simulink library "SimulationLibrary"  (R2016b)
settings: Solver=ode45  StartTime=0.0  StopTime=10.0  RelTol=1e-3  EnableMultiTasking=on
values from neighbouring files (symbols this model uses):
  cassieEtherCatData = cassieEtherCat.getStructure    [simulationInitFcn.m]
  pelvisPosition = [0; 0; 1.01]    [simulationInitFcn.m]
undefined symbols (not defined in the file or in its folder): CassieParameters, leftFootDrive, leftLegMedulla, pelvisMedulla, X, Y, Z
libraries: sm_lib x86, SimulationLibrary x30, nesl_utility x18, Contact_Forces_Lib x2
(part 1 of 3)
settings Model: Creator=Mikhail  LastModifiedBy=Mikhail
settings DataIOCC: LimitDataPoints=on
settings OptimizationCC: LifeSpan=inf
settings DebuggingCC: AllowSymbolicDim=off  SFUnexpectedBacktrackingDiag=warning  SFNoUnconditionalDefaultTransitionDiag=warning  SFExecutionAtInitializationDiag=none
settings GRTTargetCC: TargetLangStandard=C89/C90 (ANSI)  GeneratePreprocessorConditionals=Disable all
settings ConfigComp: CovMetricSettings=dw  CovHtmlReporting=on  CovSaveCumulativeToWorkspaceVar=on  CovSaveSingleToWorkspaceVar=on  CovExternalEMLEnable=off

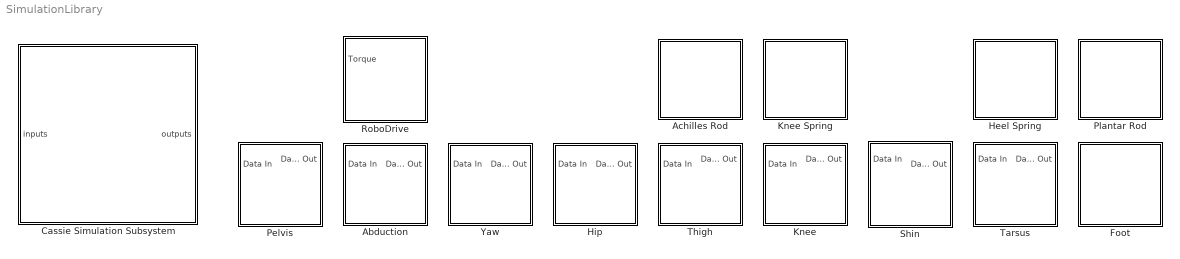
== system SimulationLibrary ==
  Abduction : Subsystem  mask{side=Left}
      mask init:
      | switch side
      |   case 1 % Left
      |     % Bus
      |     set_param([gcb, '/Bus Selector'], 'OutputSignals', 'leftAbductionDrive.outputs.torque');
      |     set_param([gcb, '/Bus Assignment'], 'AssignedSignals', 'leftAbductionDrive.inputs.position');
      |     
      |     % Solid
      |     set_param([gcb, '/Abduction'], 'ExtGeomFileName', 'left_abduction.stl');
      |     
      |     % Revolute Joint
      |     set_param([gcb, '/Revolute Joint'], 'PositionTargetValue', 'cassieEtherCatData.leftAbductionDrive.inputs.position');
      |     set_param([gcb, '/Revolute Joint'], 'DampingCoefficient', 'CassieParameters.motorViscousFrictionCoefficient(1)');
      |     
      |   case 2 % Right
      |     % Bus
      |     set_param([gcb, '/Bus Selector'], 'OutputSignals', 'rightAbductionDrive.outputs.torque');
      |     set_param([gcb, '/Bus Assignment'], 'AssignedSignals', 'rightAbductionDrive.inputs.position');
      |     
      |     % Solid
      |     set_param([gcb, '/Abduction'], 'ExtGeomFileName', 'right_abduction.stl');
      |     
      |     % Revolute Joint
      |     set_param([gcb, '/Revolute Joint'], 'PositionTargetValue', 'cassieEtherCatData.rightAbductionDrive.inputs.position');
      |     set_param([gcb, '/Revolute Joint'], 'DampingCoefficient', 'CassieParameters.motorViscousFrictionCoefficient(6)');
      | end % switch
      mask TypeOptions side: Left | Right
      mask Display: image('Cassie Abduction.png');
  Achilles Rod : Subsystem
      mask Display: image('Cassie Achilles Rod.png')
  Cassie Simulation Subsystem : Subsystem
      mask Display: image('Cassie.png');
  Foot : Subsystem  mask{side=Left}
      mask init:
      | switch side
      |   case 1 % Left
      |     % Solid
      |     set_param([gcb, '/Foot'], 'ExtGeomFileName', 'left_foot.stl');
      |     set_param([gcb, '/Foot'], 'CenterOfMass', '[4.74; 27.48; -0.14]/1000');
      |     set_param([gcb, '/Foot'], 'ProductsOfInertia', '[0.1716; -1.456; -98.63]/1000000');
      |     
      |     % Plantar
      |     set_param([gcb, '/Foot to Plantar Rod'], 'TranslationCartesianOffset', '[55; 0; 7.76]/1000');
      |     
      |     % Joint
      |     set_param([gcb, '/Revolute Joint'], 'PositionTargetValue', 'cassieEtherCatData.leftFootDrive.inputs.position');
      |     
      |   case 2 % Right
      |     % Solid
      |     set_param([gcb, '/Foot'], 'ExtGeomFileName', 'right_foot.stl');
      |     set_param([gcb, '/Foot'], 'CenterOfMass', '[4.74; 27.48; 0.14]/1000');
      |     set_param([gcb, '/Foot'], 'ProductsOfInertia', '[-0.1716; 1.456; -98.63]/1000000');
      |     
      |     % Plantar
      |     set_param([gcb, '/Foot to Plantar Rod'], 'TranslationCartesianOffset', '[55; 0; -7.76]/1000');
      |     
      |     % Joint
      |     set_param([gcb, '/Revolute Joint'], 'PositionTargetValue', 'cassieEtherCatData.rightFootDrive.inputs.position');
      | end % switch
      mask TypeOptions side: Left | Right
      mask Display: image('Cassie Foot.png');
  Heel Spring : Subsystem
  Hip : Subsystem  mask{side=Left}
      mask init:
      | switch side
      |   case 1 % Left
      |     % Bus
      |     set_param([gcb, '/Bus Selector'], 'OutputSignals', 'leftHipDrive.outputs.torque');
      |     set_param([gcb, '/Bus Assignment'], 'AssignedSignals', 'leftHipDrive.inputs.position');
      |     
      |     % Solid
      |     set_param([gcb, '/Hip'], 'ExtGeomFileName', 'left_hip.stl');
      |     set_param([gcb, '/Hip'], 'CenterOfMass', '[-55.72; 0; 0.01]/1000');
      |     set_param([gcb, '/Hip'], 'ProductsOfInertia', '[-0.04; -0.6251; 0.2462]/1000000');
      |     
      |     % Revolute Joint
      |     set_param([gcb, '/Revolute Joint'], 'PositionTargetValue', 'cassieEtherCatData.leftHipDrive.inputs.position');
      |     set_param([gcb, '/Revolute Joint'], 'DampingCoefficient', 'CassieParameters.motorViscousFrictionCoefficient(3)');
      |     
      |   case 2 % Right
      |     % Bus
      |     set_param([gcb, '/Bus Selector'], 'OutputSignals', 'rightHipDrive.outputs.torque');
      |     set_param([gcb, '/Bus Assignment'], 'AssignedSignals', 'rightHipDrive.inputs.position');
      |     
      |     % Solid
      |     set_param([gcb, '/Hip'], 'ExtGeomFileName', 'right_hip.stl');
      |     set_param([gcb, '/Hip'], 'CenterOfMass', '[-55.72; 0; -0.01]/1000');
      |     set_param([gcb, '/Hip'], 'ProductsOfInertia', '[0.04; 0.6251; 0.2462]/1000000');
      |     
      |     % Revolute Joint
      |     set_param([gcb, '/Revolute Joint'], 'PositionTargetValue', 'cassieEtherCatData.rightHipDrive.inputs.position');
      |     set_param([gcb, '/Revolute Joint'], 'DampingCoefficient', 'CassieParameters.motorViscousFrictionCoefficient(8)');
      | end % switch
      mask TypeOptions side: Left | Right
      mask Display: image('Cassie Hip.png');
  Knee : Subsystem  mask{side=Left}
      mask init:
      | switch side
      |   case 1 % Left
      |     % Bus
      |     set_param([gcb, '/Bus Selector'], 'OutputSignals', 'leftKneeDrive.outputs.torque');
      |     set_param([gcb, '/Bus Assignment'], 'AssignedSignals', 'leftKneeDrive.inputs.position');
      |     
      |     % Solid
      |     set_param([gcb, '/Knee'], 'ExtGeomFileName', 'left_knee.stl');
      |     set_param([gcb, '/Knee'], 'CenterOfMass', '[23.0; 32.07; -2.181]/1000');
      |     set_param([gcb, '/Knee'], 'ProductsOfInertia', '[0.739; 2.837; 956.4]/1000000');
      |     
      |     % Revolute Joint
      |     set_param([gcb, '/Revolute Joint'], 'PositionTargetValue', 'cassieEtherCatData.leftKneeDrive.inputs.position');
      |     set_param([gcb, '/Revolute Joint'], 'DampingCoefficient', 'CassieParameters.motorViscousFrictionCoefficient(4)');
      |     
      |   case 2 % Right
      |     % Bus
      |     set_param([gcb, '/Bus Selector'], 'OutputSignals', 'rightKneeDrive.outputs.torque');
      |     set_param([gcb, '/Bus Assignment'], 'AssignedSignals', 'rightKneeDrive.inputs.position');
      |     
      |     % Solid
      |     set_param([gcb, '/Knee'], 'ExtGeomFileName', 'right_knee.stl');
      |     set_param([gcb, '/Knee'], 'CenterOfMass', '[23.0; 32.07; 2.181]/1000');
      |     set_param([gcb, '/Knee'], 'ProductsOfInertia', '[-0.739; -2.837; 956.4]/1000000');
      |     
      |     % Revolute Joint
      |     set_param([gcb, '/Revolute Joint'], 'PositionTargetValue', 'cassieEtherCatData.rightKneeDrive.inputs.position');
      |     set_param([gcb, '/Revolute Joint'], 'DampingCoefficient', 'CassieParameters.motorViscousFrictionCoefficient(9)');
      | end % switch
      mask TypeOptions side: Left | Right
      mask Display: image('Cassie Knee.png');
  Knee Spring : Subsystem
  Pelvis : Subsystem
      mask Display: image('Cassie Pelvis.png');
  Plantar Rod : Subsystem
      mask Display: image('Cassie Plantar Rod.png')
  RoboDrive : Subsystem  mask{model=115x25}
      mask prompts: model "RoboDrive model:"
      mask init:
      | switch model
      |   case 1 % 115x25
      |     set_param([gcb '/Peak Torque'], 'Value', '12.2');
      |     set_param([gcb '/Peak Speed'], 'Value', '1300*2*pi/60');
      |     set_param([gcb '/Rotor'], 'MomentsOfInertia', '[0 0 365]/1000000');
      |   case 2 % 85x13
      |     set_param([gcb '/Peak Torque'], 'Value', '4.5');
      |     set_param([gcb '/Peak Speed'], 'Value', '2900*2*pi/60');
      |     set_param([gcb '/Rotor'], 'MomentsOfInertia', '[0 0 61]/1000000');
      |   case 3 % 50x8
      |     set_param([gcb '/Peak Torque'], 'Value', '0.9');
      |     set_param([gcb '/Peak Speed'], 'Value', '5500*2*pi/60');
      |     set_param([gcb '/Rotor'], 'MomentsOfInertia', '[0 0 4.9]/1000000');
      | end % switch
      mask TypeOptions model: 115x25 | 85x13 | 50x8
      mask Display: image('RoboDrive.png')
  Shin : Subsystem  mask{side=Left}
      mask init:
      | switch side
      |   case 1 % Left
      |     % Bus
      |     set_param([gcb, '/Bus Assignment'], 'AssignedSignals', 'leftLegMedulla.miscInputs.kneeSpringEncoder');
      |     
      |     % Solid
      |     set_param([gcb, '/Shin'], 'ExtGeomFileName', 'left_shin.stl');
      |     set_param([gcb, '/Shin'], 'CenterOfMass', '[183.38; 1.169; 0.2123]/1000');
      |     set_param([gcb, '/Shin'], 'ProductsOfInertia', '[0.2652; -0.1941; 333.5]/1000000');
      |     
      |   case 2 % Right
      |     % Bus
      |     set_param([gcb, '/Bus Assignment'], 'AssignedSignals', 'rightLegMedulla.miscInputs.kneeSpringEncoder');
      |     
      |     % Solid
      |     set_param([gcb, '/Shin'], 'ExtGeomFileName', 'right_shin.stl');
      |     set_param([gcb, '/Shin'], 'CenterOfMass', '[183.38; 1.169; -0.2123]/1000');
      |     set_param([gcb, '/Shin'], 'ProductsOfInertia', '[-0.2652; 0.1941; 333.5]/1000000');
      | end % switch
      mask TypeOptions side: Left | Right
      mask Display: image('Cassie Shin.png');
  Tarsus : Subsystem  mask{side=Left}
      mask init:
      | switch side
      |   case 1 % Left
      |     % Bus
      |     set_param([gcb, '/Bus Selector'], 'OutputSignals', 'leftFootDrive.outputs.torque');
      |     set_param([gcb, '/Bus Assignment'], 'AssignedSignals', 'leftFootDrive.inputs.position,leftLegMedulla.miscInputs.ankleJointEncoder');
      |     
      |     % Solid
      |     set_param([gcb, '/Tarsus'], 'ExtGeomFileName', 'left_tarsus.stl');
      |     set_param([gcb, '/Tarsus'], 'CenterOfMass', '[110.46; -30.58; -1.31]/1000');
      |     set_param([gcb, '/Tarsus'], 'ProductsOfInertia', '[36.15; -63.29; -2878]/1000000');
      |     
      |     % Transforms
      |     set_param([gcb, '/Tarsus to Foot Drive'], 'TranslationCartesianOffset', '[58 -34 22.75]/1000');
      |     set_param([gcb, '/Tarsus to Spring'], 'TranslationCartesianOffset', '[-12.69 -30.59 0.92]/1000');
      |     set_param([gcb, '/Tarsus to Spring'], 'RotationSequenceAngles', '[155.8, 0.315, 4.47]');
      |     set_param([gcb, '/Foot Crank to Plantar Rod'], 'TranslationCartesianOffset', '[55 0 -7.91]/1000');
      |     set_param([gcb, '/Foot Crank Transform'], 'RotationAngle', '0');
      |     
      |     % Revolute Joint
      |     set_param([gcb, '/Foot Crank Revolute Joint'], 'PositionTargetValue', 'cassieEtherCatData.leftFootDrive.inputs.position');
      |     set_param([gcb, '/Foot Crank Revolute Joint'], 'DampingCoefficient', 'CassieParameters.motorViscousFrictionCoefficient(5)');
      |     
      |   case 2 % Right
      |     % Bus
      |     set_param([gcb, '/Bus Selector'], 'OutputSignals', 'rightFootDrive.outputs.torque');
      |     set_param([gcb, '/Bus Assignment'], 'AssignedSignals', 'rightFootDrive.inputs.position,rightLegMedulla.miscInputs.ankleJointEncoder');
      |     
      |     % Solid
      |     set_param([gcb, '/Tarsus'], 'ExtGeomFileName', 'right_tarsus.stl');
      |     set_param([gcb, '/Tarsus'], 'CenterOfMass', '[110.46; -30.58; 1.31]/1000');
      |     set_param([gcb, '/Tarsus'], 'ProductsOfInertia', '[-36.15; 63.29; -2878]/1000000');
      |     
      |     % Transforms
      |     set_param([gcb, '/Tarsus to Foot Drive'], 'TranslationCartesianOffset', '[58 -34 -22.75]/1000');
      |     set_param([gcb, '/Tarsus to Spring'], 'TranslationCartesianOffset', '[-12.69 -30.59 -0.92]/1000');
      |     set_param([gcb, '/Tarsus to Spring'], 'RotationSequenceAngles', '[155.8, -0.315, -4.47]');
      |     set_param([gcb, '/Foot Crank to Plantar Rod'], 'TranslationCartesianOffset', '[55 0 7.91]/1000');
      |     set_param([gcb, '/Foot Crank Transform'], 'RotationAngle', 'pi');
      |     
      |     % Revolute Joint
      |     set_param([gcb, '/Foot Crank Revolute Joint'], 'PositionTargetValue', 'cassieEtherCatData.rightFootDrive.inputs.position');
      |     set_param([gcb, '/Foot Crank Revolute Joint'], 'DampingCoefficient', 'CassieParameters.motorViscousFrictionCoefficient(10)');
      | end % switch
      mask TypeOptions side: Left | Right
      mask Display: image('Cassie Tarsus.png');
  Thigh : Subsystem  mask{side=Left}
      mask init:
      | switch side
      |   case 1 % Left
      |     % Solid
      |     set_param([gcb, '/Thigh'], 'ExtGeomFileName', 'left_thigh.stl');
      |     set_param([gcb, '/Thigh'], 'CenterOfMass', '[59.46; 0.05; -35.81]/1000');
      |     set_param([gcb, '/Thigh'], 'ProductsOfInertia', '[-19.26; -11685; 283.6]/1000000');
      |     
      |     % Knee
      |     set_param([gcb, '/Thigh to Knee'], 'TranslationCartesianOffset', '[0.12, 0, 0.0045]');
      |     
      |     % Achilles
      |     set_param([gcb, '/Thigh to Achilles'], 'TranslationCartesianOffset', '[0, 0, 0.045]');
      |     
      |   case 2 % Right
      |     % Solid
      |     set_param([gcb, '/Thigh'], 'ExtGeomFileName', 'right_thigh.stl');
      |     set_param([gcb, '/Thigh'], 'CenterOfMass', '[59.46; 0.05; 35.81]/1000');
      |     set_param([gcb, '/Thigh'], 'ProductsOfInertia', '[19.26; 11685; 283.6]/1000000');
      |     
      |     % Knee
      |     set_param([gcb, '/Thigh to Knee'], 'TranslationCartesianOffset', '[0.12, 0, -0.0045]');
      |     
      |     % Achilles
      |     set_param([gcb, '/Thigh to Achilles'], 'TranslationCartesianOffset', '[0, 0, -0.045]');
      | end % switch
      mask TypeOptions side: Left | Right
      mask Display: image('Cassie Thigh.png');
  Yaw : Subsystem  mask{side=Left}
      mask init:
      | switch side
      |   case 1 % Left
      |     % Bus
      |     set_param([gcb, '/Bus Selector'], 'OutputSignals', 'leftYawDrive.outputs.torque');
      |     set_param([gcb, '/Bus Assignment'], 'AssignedSignals', 'leftYawDrive.inputs.position');
      |     
      |     % Solid
      |     set_param([gcb, '/Yaw'], 'ExtGeomFileName', 'left_yaw.stl');
      |     set_param([gcb, '/Yaw'], 'CenterOfMass', '[25.7; 0.1; 17.93]/1000');
      |     set_param([gcb, '/Yaw'], 'ProductsOfInertia', '[2.61; 1.53; 0.703]/1000000');
      |     
      |     % Revolute Joint
      |     set_param([gcb, '/Revolute Joint'], 'PositionTargetValue', 'cassieEtherCatData.leftYawDrive.inputs.position');
      |     set_param([gcb, '/Revolute Joint'], 'DampingCoefficient', 'CassieParameters.motorViscousFrictionCoefficient(2)');
      |     
      |   case 2 % Right
      |     % Bus
      |     set_param([gcb, '/Bus Selector'], 'OutputSignals', 'rightYawDrive.outputs.torque');
      |     set_param([gcb, '/Bus Assignment'], 'AssignedSignals', 'rightYawDrive.inputs.position');
      |     
      |     % Solid
      |     set_param([gcb, '/Yaw'], 'ExtGeomFileName', 'right_yaw.stl');
      |     set_param([gcb, '/Yaw'], 'CenterOfMass', '[25.7; -0.1; 17.93]/1000');
      |     set_param([gcb, '/Yaw'], 'ProductsOfInertia', '[-2.61; 1.53; -0.703]/1000000');
      |     
      |     % Revolute Joint
      |     set_param([gcb, '/Revolute Joint'], 'PositionTargetValue', 'cassieEtherCatData.rightYawDrive.inputs.position');
      |     set_param([gcb, '/Revolute Joint'], 'DampingCoefficient', 'CassieParameters.motorViscousFrictionCoefficient(7)');
      | end % switch
      mask TypeOptions side: Left | Right
      mask Display: image('Cassie Yaw.png');

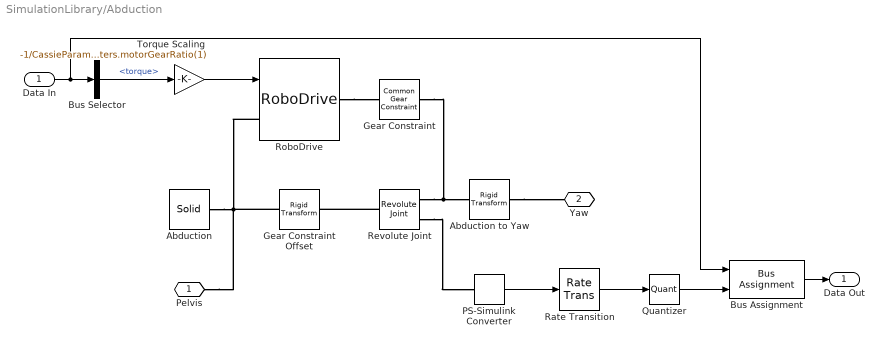
== system SimulationLibrary/Abduction ==
  Data In : Inport  OutDataTypeStr=Bus: cassieEtherCatBus
  Abduction : sm_lib/Body Elements/Solid  InertiaType=Custom  Mass=0  MassUnits=kg  CenterOfMass=[0; 0; 0]  CenterOfMassUnits=m  MomentsOfInertia=[0; 0; 0]  MomentsOfInertiaUnits=kg*m^2  ProductsOfInertia=[0; 0; 0]  ProductsOfInertiaUnits=kg*m^2  DensityBased=on  Density=1000  DensityUnits=kg/(m^3)  DoExposeReferenceFrame=on  SerializedFrames=<Frames/>  GraphicType=FromGeometry  MarkerShape=Sphere  MarkerSize=10  MarkerSizeUnits=m  GraphicVisPropType=AdvancedVisualProperties  GraphicDiffuseColor=simulationParameters.diffuseColor  GraphicSpecularColor=simulationParameters.specularColor  GraphicAmbientColor=simulationParameters.ambientColor  GraphicEmissiveColor=simulationParameters.emissiveColor  GraphicShininess=simulationParameters.shininess  GraphicOpacity=1  GeometryShape=FromFile  RectangleSize=[1 1]  RectangleSizeUnits=m  BrickDimensions=[0.15 0.15 0.2]  BrickDimensionUnits=m  CylinderRadius=0.05  CylinderRadiusUnits=m  CylinderLength=0.1  CylinderLengthUnits=m  SphereRadius=1  SphereRadiusUnits=m  EllipsoidRadii=[1 1 1]  EllipsoidRadiiUnits=m  ExtrusionCrossSection=[1 1; -1 1; -1 -1; 1 -1]  ExtrusionCrossSectionUnits=m  ExtrusionLength=1  ExtrusionLengthUnits=m  PolygonNumSides=3  PolygonOuterRadius=1  PolygonOuterRadiusUnits=m  ExtGeomFileType=STL  ExtGeomFileName=left_abduction.stl  ExtGeomFileUnits=m  RevolutionCrossSection=[1 1; 1 -1; 2 -1; 2 1]  RevolutionCrossSectionUnits=m  RevolutionExtent=Full  RevolutionAngle=180  RevolutionAngleUnits=deg
  Abduction to Yaw : sm_lib/Frames and Transforms/Rigid Transform  TranslationMethod=Cartesian  TranslationStandardOffset=0  TranslationLengthUnit=m  TranslationStandardAxis=+Z  TranslationCartesianOffset=[0, 0, -0.07]  TranslationROffset=0  TranslationROffsetUnits=m  TranslationZOffset=0  TranslationZOffsetUnits=m  TranslationThetaOffset=0  TranslationThetaOffsetUnits=deg  RotationMethod=RotationMatrix  RotationAngleUnits=deg  RotationStandardAxis=+Z  RotationAngle=0.0  RotationArbitraryAxis=[0 0 1]  FollAlignAxisA=+X  BaseAlignAxisA=+Y  FollAlignAxisB=+Y  BaseAlignAxisB=+Z  RotationSequenceAxes=FollowerAxes  RotationSequence=XYZ  RotationSequenceAngles=[90 0 0]  RotationSequenceAnglesUnits=deg  RotationMatrix=[0, 0, -1; 0, 1, 0; 1, 0, 0]
  Bus Assignment : BusAssignment  AssignedSignals=leftAbductionDrive.inputs.position
  Bus Selector : BusSelector  OutputSignals=leftAbductionDrive.outputs.torque
  Gear Constraint : sm_lib/Gears and Couplings/Gears/Common Gear Constraint  GearType=External  SpecificationType=CenterDistanceRatio  CenterDistance=1e-6  CenterDistanceUnits=m  GearRatio=CassieParameters.motorGearRatio(1)  BaseGearRadius=10.0  BaseGearRadiusUnits=cm  FollGearRadius=10.0  FollGearRadiusUnits=cm  AssemblyGearRotation=Free
  Gear Constraint Offset : sm_lib/Frames and Transforms/Rigid Transform  TranslationMethod=StandardAxis  TranslationStandardOffset=1e-6  TranslationLengthUnit=m  TranslationStandardAxis=+Y  TranslationCartesianOffset=[0 0 0]  TranslationROffset=0  TranslationROffsetUnits=m  TranslationZOffset=0  TranslationZOffsetUnits=m  TranslationThetaOffset=0  TranslationThetaOffsetUnits=deg  RotationMethod=None  RotationAngleUnits=deg  RotationStandardAxis=+Z  RotationAngle=0.0  RotationArbitraryAxis=[0 0 1]  FollAlignAxisA=+X  BaseAlignAxisA=+Y  FollAlignAxisB=+Y  BaseAlignAxisB=+Z  RotationSequenceAxes=FollowerAxes  RotationSequence=XYX  RotationSequenceAngles=[0 0 0]  RotationSequenceAnglesUnits=deg  RotationMatrix=[1 0 0; 0 1 0; 0 0 1]
  PS-Simulink Converter : nesl_utility/PS-Simulink Converter  PhysicalDomain=network_engine_domain  SubClassName=ps_output  LeftPortType=input  RightPortType=output  PseudoPeriodic=off  Frequencies=[]  Unit=rad  AffineConversion=off
  Quantizer : Quantizer  QuantizationInterval=(2*pi)/(CassieParameters.motorEncoderTicks(1)*CassieParameters.motorGearRatio(1))
  Rate Transition : RateTransition  Deterministic=off  OutPortSampleTime=CassieParameters.etherCatSampleTime
  Revolute Joint : sm_lib/Joints/Revolute Joint  SenseConstraintForce=off  SenseConstraintForceX=off  SenseConstraintForceY=off  SenseConstraintForceZ=off  SenseConstraintTorque=off  SenseConstraintTorqueX=off  SenseConstraintTorqueY=off  SenseConstraintTorqueZ=off  SenseTotalForce=off  SenseTotalForceX=off  SenseTotalForceY=off  SenseTotalForceZ=off  SenseTotalTorque=off  SenseTotalTorqueX=off  SenseTotalTorqueY=off  SenseTotalTorqueZ=off  CompositeWrenchDir=FollowerOnBase  CompositeWrenchFrame=BaseFrame  EquilibriumPosition=0  EquilibriumPositionUnits=rad  SpringStiffness=0  SpringStiffnessUnits=N*m/rad  DampingCoefficient=CassieParameters.motorViscousFrictionCoefficient(1)  DampingCoefficientUnits=N*m/(rad/s)  TorqueActuationMode=NoTorque  MotionActuationMode=ComputedMotion  SensePosition=on  SenseVelocity=off  SenseAcceleration=off  SenseTorqueForce=off  PositionTargetSpecify=on  PositionTargetPriority=High  PositionTargetValue=cassieEtherCatData.leftAbductionDrive.inputs.position  PositionTargetValueUnits=rad  VelocityTargetSpecify=on  VelocityTargetPriority=High  VelocityTargetValue=0  VelocityTargetValueUnits=rad/s
  RoboDrive : SimulationLibrary/RoboDrive  model=85x13
  Torque Scaling : Gain  Gain=-1/CassieParameters.motorGearRatio(1)
  Pelvis : PMIOPort  Port=1  Side=Left
  Yaw : PMIOPort  Port=2  Side=Right
  Data Out : Outport
  wires:
  Torque Scaling/1 -> RoboDrive/1
  Data In/1 -> Bus Selector/1, Bus Assignment/1
  Bus Assignment/1 -> Data Out/1
  Rate Transition/1 -> Quantizer/1
  Bus Selector/1 -> Torque Scaling/1  "<torque>"
  PS-Simulink Converter/1 -> Rate Transition/1
  Quantizer/1 -> Bus Assignment/2
  connections:
  Pelvis/RConn1 -- RoboDrive/LConn1 -- Abduction/RConn1 -- Gear Constraint Offset/LConn1
  Revolute Joint/LConn1 -- Gear Constraint Offset/RConn1
  RoboDrive/RConn1 -- Gear Constraint/LConn1
  Revolute Joint/RConn1 -- Abduction to Yaw/LConn1 -- Gear Constraint/RConn1
  Revolute Joint/RConn2 -- PS-Simulink Converter/LConn1
  Abduction to Yaw/RConn1 -- Yaw/RConn1

== system SimulationLibrary/Achilles Rod ==
  Achilles Rod : sm_lib/Body Elements/Solid  Commented=on  InertiaType=Custom  Mass=0.1567  MassUnits=kg  CenterOfMass=[247.19; 0; 0]/1000  CenterOfMassUnits=m  MomentsOfInertia=[3.7538; 14061; 14061]/1000000  MomentsOfInertiaUnits=kg*m^2  ProductsOfInertia=[0; 0.0082; 0.0068]/1000000  ProductsOfInertiaUnits=kg*m^2  DensityBased=on  Density=1000  DensityUnits=kg/(m^3)  DoExposeReferenceFrame=on  SerializedFrames=<Frames/>  GraphicType=FromGeometry  MarkerShape=Sphere  MarkerSize=10  GraphicVisPropType=AdvancedVisualProperties  GraphicDiffuseColor=simulationParameters.diffuseColor  GraphicSpecularColor=simulationParameters.specularColor  GraphicAmbientColor=simulationParameters.ambientColor  GraphicEmissiveColor=simulationParameters.emissiveColor  GraphicShininess=simulationParameters.shininess  GraphicOpacity=1.0  GeometryShape=FromFile  RectangleSize=[1 1]  RectangleSizeUnits=m  BrickDimensions=[1 1 1]  BrickDimensionUnits=m  CylinderRadius=1  CylinderRadiusUnits=m  CylinderLength=1  CylinderLengthUnits=m  SphereRadius=1  SphereRadiusUnits=m  EllipsoidRadii=[1 1 1]  EllipsoidRadiiUnits=m  ExtrusionCrossSection=[1 1; -1 1; -1 -1; 1 -1]  ExtrusionCrossSectionUnits=m  ExtrusionLength=1  ExtrusionLengthUnits=m  PolygonNumSides=3  PolygonOuterRadius=1  PolygonOuterRadiusUnits=m  ExtGeomFileType=STL  ExtGeomFileName=achilles_rod.stl  ExtGeomFileUnits=m  RevolutionCrossSection=[1 1; 1 -1; 2 -1; 2 1]  RevolutionCrossSectionUnits=m  RevolutionExtent=Full  RevolutionAngle=180  RevolutionAngleUnits=deg
  Distance Constraint : sm_lib/Constraints/Distance Constraint  Distance=0.5012  DistanceUnits=m  SenseSignedForceMagnitude=off  SenseTorque=off  SenseForce=off  WrenchDir=FollowerOnBase  WrenchFrame=BaseFrame
  Rigid Transform : sm_lib/Frames and Transforms/Rigid Transform  Commented=on  TranslationMethod=Cartesian  TranslationStandardOffset=50.14  TranslationLengthUnit=m  TranslationStandardAxis=+Z  TranslationCartesianOffset=[0.5012 0 0]  TranslationROffset=0  TranslationROffsetUnits=m  TranslationZOffset=0  TranslationZOffsetUnits=m  TranslationThetaOffset=0  TranslationThetaOffsetUnits=deg  RotationMethod=None  RotationAngleUnits=deg  RotationStandardAxis=+Z  RotationAngle=0.0  RotationArbitraryAxis=[0 0 1]  FollAlignAxisA=+X  BaseAlignAxisA=+Y  FollAlignAxisB=+Y  BaseAlignAxisB=+Z  RotationSequenceAxes=FollowerAxes  RotationSequence=XYX  RotationSequenceAngles=[0 0 0]  RotationSequenceAnglesUnits=deg  RotationMatrix=[1 0 0; 0 1 0; 0 0 1]
  Spring Spherical Joint : sm_lib/Joints/Spherical Joint  Commented=on  SenseConstraintForce=off  SenseConstraintForceX=off  SenseConstraintForceY=off  SenseConstraintForceZ=off  SenseConstraintTorque=off  SenseConstraintTorqueX=off  SenseConstraintTorqueY=off  SenseConstraintTorqueZ=off  SenseTotalForce=off  SenseTotalForceX=off  SenseTotalForceY=off  SenseTotalForceZ=off  SenseTotalTorque=off  SenseTotalTorqueX=off  SenseTotalTorqueY=off  SenseTotalTorqueZ=off  CompositeWrenchDir=FollowerOnBase  CompositeWrenchFrame=BaseFrame  DefPosRotationMethod=None  DefPosRotationAngleUnits=deg  DefPosRotationStandardAxis=+Z  DefPosRotationAngle=0.0  DefPosRotationArbitraryAxis=[0 0 1]  DefPosFollAlignAxisA=+X  DefPosBaseAlignAxisA=+Y  DefPosFollAlignAxisB=+Y  DefPosBaseAlignAxisB=+Z  DefPosRotationSequenceAxes=FollowerAxes  DefPosRotationSequence=XYX  DefPosRotationSequenceAngles=[0 0 0]  DefPosRotationSequenceAnglesUnits=deg  DefPosRotationMatrix=[1 0 0; 0 1 0; 0 0 1]  EqPosRotationMethod=None  EqPosRotationAngleUnits=deg  EqPosRotationStandardAxis=+Z  EqPosRotationAngle=0.0  EqPosRotationArbitraryAxis=[0 0 1]  EqPosFollAlignAxisA=+X  EqPosBaseAlignAxisA=+Y  EqPosFollAlignAxisB=+Y  EqPosBaseAlignAxisB=+Z  EqPosRotationSequenceAxes=FollowerAxes  EqPosRotationSequence=XYX  EqPosRotationSequenceAngles=[0 0 0]  EqPosRotationSequenceAnglesUnits=deg  EqPosRotationMatrix=[1 0 0; 0 1 0; 0 0 1]  SpringStiffness=0  SpringStiffnessUnits=N*m/deg  DampingCoefficient=0  DampingCoefficientUnits=N*m/(deg/s)  ActuateTorqueX=off  ActuateTorqueY=off  ActuateTorqueZ=off  ActuateTorque=off  TorqueActuationMode=NoTorque  MotionActuationMode=ComputedMotion  ActuationFrame=BaseFrame  SensePosition=off  SenseVelocityX=off  SenseVelocityY=off  SenseVelocityZ=off  SenseVelocity=off  SenseAccelerationX=off  SenseAccelerationY=off  SenseAccelerationZ=off  SenseAcceleration=off  SenseTorqueX=off  SenseTorqueY=off  SenseTorqueZ=off  SenseTorqueForce=off  SensingFrame=BaseFrame  PositionTargetRotationMethod=None  PositionTargetRotationAngleUnits=deg  PositionTargetRotationStandardAxis=+Z  PositionTargetRotationAngle=0.0  PositionTargetRotationArbitraryAxis=[0 0 1]  PositionTargetFollAlignAxisA=+X  PositionTargetBaseAlignAxisA=+Y  PositionTargetFollAlignAxisB=+Y  PositionTargetBaseAlignAxisB=+Z  PositionTargetRotationSequenceAxes=FollowerAxes  PositionTargetRotationSequence=XYX  PositionTargetRotationSequenceAngles=[0 0 0]  PositionTargetRotationSequenceAnglesUnits=deg  PositionTargetRotationMatrix=[1 0 0; 0 1 0; 0 0 1]  PositionTargetSpecify=off  PositionTargetPriority=High  VelocityTargetValue=[0 0 0]  VelocityTargetValueUnits=deg/s  VelocityTargetSpecify=off  VelocityTargetPriority=High  VelocityTargetInFollowerFrame=on
  Thigh Spherical Joint : sm_lib/Joints/Spherical Joint  Commented=on  SenseConstraintForce=off  SenseConstraintForceX=off  SenseConstraintForceY=off  SenseConstraintForceZ=off  SenseConstraintTorque=off  SenseConstraintTorqueX=off  SenseConstraintTorqueY=off  SenseConstraintTorqueZ=off  SenseTotalForce=off  SenseTotalForceX=off  SenseTotalForceY=off  SenseTotalForceZ=off  SenseTotalTorque=off  SenseTotalTorqueX=off  SenseTotalTorqueY=off  SenseTotalTorqueZ=off  CompositeWrenchDir=FollowerOnBase  CompositeWrenchFrame=BaseFrame  DefPosRotationMethod=None  DefPosRotationAngleUnits=deg  DefPosRotationStandardAxis=+Z  DefPosRotationAngle=0.0  DefPosRotationArbitraryAxis=[0 0 1]  DefPosFollAlignAxisA=+X  DefPosBaseAlignAxisA=+Y  DefPosFollAlignAxisB=+Y  DefPosBaseAlignAxisB=+Z  DefPosRotationSequenceAxes=FollowerAxes  DefPosRotationSequence=XYX  DefPosRotationSequenceAngles=[0 0 0]  DefPosRotationSequenceAnglesUnits=deg  DefPosRotationMatrix=[1 0 0; 0 1 0; 0 0 1]  EqPosRotationMethod=None  EqPosRotationAngleUnits=deg  EqPosRotationStandardAxis=+Z  EqPosRotationAngle=0.0  EqPosRotationArbitraryAxis=[0 0 1]  EqPosFollAlignAxisA=+X  EqPosBaseAlignAxisA=+Y  EqPosFollAlignAxisB=+Y  EqPosBaseAlignAxisB=+Z  EqPosRotationSequenceAxes=FollowerAxes  EqPosRotationSequence=XYX  EqPosRotationSequenceAngles=[0 0 0]  EqPosRotationSequenceAnglesUnits=deg  EqPosRotationMatrix=[1 0 0; 0 1 0; 0 0 1]  SpringStiffness=0  SpringStiffnessUnits=N*m/deg  DampingCoefficient=0  DampingCoefficientUnits=N*m/(deg/s)  ActuateTorqueX=off  ActuateTorqueY=off  ActuateTorqueZ=off  ActuateTorque=off  TorqueActuationMode=NoTorque  MotionActuationMode=ComputedMotion  ActuationFrame=BaseFrame  SensePosition=off  SenseVelocityX=off  SenseVelocityY=off  SenseVelocityZ=off  SenseVelocity=off  SenseAccelerationX=off  SenseAccelerationY=off  SenseAccelerationZ=off  SenseAcceleration=off  SenseTorqueX=off  SenseTorqueY=off  SenseTorqueZ=off  SenseTorqueForce=off  SensingFrame=BaseFrame  PositionTargetRotationMethod=None  PositionTargetRotationAngleUnits=deg  PositionTargetRotationStandardAxis=+Z  PositionTargetRotationAngle=0.0  PositionTargetRotationArbitraryAxis=[0 0 1]  PositionTargetFollAlignAxisA=+X  PositionTargetBaseAlignAxisA=+Y  PositionTargetFollAlignAxisB=+Y  PositionTargetBaseAlignAxisB=+Z  PositionTargetRotationSequenceAxes=FollowerAxes  PositionTargetRotationSequence=XYX  PositionTargetRotationSequenceAngles=[0 0 0]  PositionTargetRotationSequenceAnglesUnits=deg  PositionTargetRotationMatrix=[1 0 0; 0 1 0; 0 0 1]  PositionTargetSpecify=off  PositionTargetPriority=High  VelocityTargetValue=[0 0 0]  VelocityTargetValueUnits=deg/s  VelocityTargetSpecify=off  VelocityTargetPriority=High  VelocityTargetInFollowerFrame=on
  Thigh : PMIOPort  Port=1  Side=Left
  Heel Spring : PMIOPort  Port=2  Side=Right
  connections:
  Distance Constraint/LConn1 -- Thigh/RConn1
  Distance Constraint/RConn1 -- Heel Spring/RConn1
  Achilles Rod/RConn1 -- Thigh Spherical Joint/RConn1 -- Rigid Transform/LConn1
  Spring Spherical Joint/LConn1 -- Rigid Transform/RConn1

== system SimulationLibrary/Cassie Simulation Subsystem ==
  inputs : Inport  OutDataTypeStr=Bus: cassieInputsBus  PortDimensions=[1 1]  SampleTime=CassieParameters.etherCatSampleTime  BusOutputAsStruct=on
  Cassie Inputs Processing MATLAB System : MATLABSystem  System=ProcessInputsSimulation  SimulateUsing=Code generation
      mask Type: ProcessInputsSimulation
      mask Display:
      | disp('ProcessInputsSimulation');
      | port_label('input',1,'etherCat');
      | port_label('input',2,'inputs');
      | port_label('input',3,'outputs');
      | port_label('output',1,'etherCat');
  Cassie Multibody Subsystem : Subsystem
      mask Display: image('Cassie.png');
  Cassie Outputs Processing MATLAB System : MATLABSystem  System=ProcessOutputsSimulation  SimulateUsing=Code generation
      mask Type: ProcessOutputsSimulation
      mask Display:
      | disp('ProcessOutputsSimulation');
      | port_label('input',1,'etherCat');
      | port_label('output',1,'etherCat');
      | port_label('output',2,'outputs');
  EtherCAT Delay : Delay  DelayLength=1  InitialCondition=cassieEtherCatData  InputProcessing=Inherited
  Outputs Delay : Delay  DelayLength=1  InputProcessing=Inherited
  outputs : Outport  OutDataTypeStr=Bus: cassieOutputsBus  PortDimensions=[1 1]  SampleTime=CassieParameters.etherCatSampleTime  BusOutputAsStruct=on
  wires:
  Cassie Inputs Processing MATLAB System/1 -> Cassie Multibody Subsystem/1(Data In)
  Cassie Multibody Subsystem/1(Data Out) -> Cassie Outputs Processing MATLAB System/1
  Cassie Outputs Processing MATLAB System/1 -> EtherCAT Delay/1
  inputs/1 -> Cassie Inputs Processing MATLAB System/2
  EtherCAT Delay/1 -> Cassie Inputs Processing MATLAB System/1
  Outputs Delay/1 -> Cassie Inputs Processing MATLAB System/3
  Cassie Outputs Processing MATLAB System/2 -> outputs/1, Outputs Delay/1

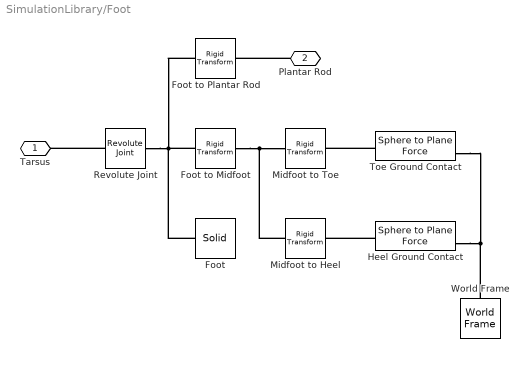
== system SimulationLibrary/Foot ==
  Foot : sm_lib/Body Elements/Solid  InertiaType=Custom  Mass=0.1498  MassUnits=kg  CenterOfMass=[4.74; 27.48; -0.14]/1000  CenterOfMassUnits=m  MomentsOfInertia=[287; 171.3; 449.1]/1000000  MomentsOfInertiaUnits=kg*m^2  ProductsOfInertia=[0.1716; -1.456; -98.63]/1000000  ProductsOfInertiaUnits=kg*m^2  DensityBased=on  Density=1000  DensityUnits=kg/(m^3)  DoExposeReferenceFrame=on  SerializedFrames=<Frames/>  GraphicType=FromGeometry  MarkerShape=Sphere  MarkerSize=10  GraphicVisPropType=AdvancedVisualProperties  GraphicDiffuseColor=simulationParameters.diffuseColor  GraphicSpecularColor=simulationParameters.specularColor  GraphicAmbientColor=simulationParameters.ambientColor  GraphicEmissiveColor=simulationParameters.emissiveColor  GraphicShininess=simulationParameters.shininess  GraphicOpacity=1  GeometryShape=FromFile  RectangleSize=[1 1]  RectangleSizeUnits=m  BrickDimensions=[0.15 0.01 0.02]  BrickDimensionUnits=m  CylinderRadius=1  CylinderRadiusUnits=m  CylinderLength=1  CylinderLengthUnits=m  SphereRadius=1  SphereRadiusUnits=m  EllipsoidRadii=[1 1 1]  EllipsoidRadiiUnits=m  ExtrusionCrossSection=[1 1; -1 1; -1 -1; 1 -1]  ExtrusionCrossSectionUnits=m  ExtrusionLength=1  ExtrusionLengthUnits=m  PolygonNumSides=3  PolygonOuterRadius=1  PolygonOuterRadiusUnits=m  ExtGeomFileType=STL  ExtGeomFileName=left_foot.stl  ExtGeomFileUnits=m  RevolutionCrossSection=[1 1; 1 -1; 2 -1; 2 1]  RevolutionCrossSectionUnits=m  RevolutionExtent=Full  RevolutionAngle=180  RevolutionAngleUnits=deg
  Foot to Midfoot : sm_lib/Frames and Transforms/Rigid Transform  TranslationMethod=Cartesian  TranslationStandardOffset=0  TranslationLengthUnit=m  TranslationStandardAxis=+Z  TranslationCartesianOffset=[17.62 52.19 0]/1000  TranslationROffset=0  TranslationROffsetUnits=m  TranslationZOffset=0  TranslationZOffsetUnits=m  TranslationThetaOffset=0  TranslationThetaOffsetUnits=deg  RotationMethod=RotationSequence  RotationAngleUnits=deg  RotationStandardAxis=+Z  RotationAngle=0.0  RotationArbitraryAxis=[0 0 1]  FollAlignAxisA=+X  BaseAlignAxisA=+Y  FollAlignAxisB=+Y  BaseAlignAxisB=+Z  RotationSequenceAxes=FollowerAxes  RotationSequence=ZYX  RotationSequenceAngles=[140 0 -90]  RotationSequenceAnglesUnits=deg  RotationMatrix=[1 0 0; 0 1 0; 0 0 1]
  Foot to Plantar Rod : sm_lib/Frames and Transforms/Rigid Transform  TranslationMethod=Cartesian  TranslationStandardOffset=0  TranslationLengthUnit=m  TranslationStandardAxis=+Z  TranslationCartesianOffset=[55; 0; 7.76]/1000  TranslationROffset=0  TranslationROffsetUnits=m  TranslationZOffset=0  TranslationZOffsetUnits=m  TranslationThetaOffset=0  TranslationThetaOffsetUnits=deg  RotationMethod=None  RotationAngleUnits=deg  RotationStandardAxis=+Z  RotationAngle=0.0  RotationArbitraryAxis=[0 0 1]  FollAlignAxisA=+X  BaseAlignAxisA=+Y  FollAlignAxisB=+Y  BaseAlignAxisB=+Z  RotationSequenceAxes=FollowerAxes  RotationSequence=XYZ  RotationSequenceAngles=[0 0 0]  RotationSequenceAnglesUnits=deg  RotationMatrix=[1 0 0; 0 1 0; 0 0 1]
  Heel Ground Contact : Contact_Forces_Lib/3D/Sphere to Plane Force  sphere_rad=0.01  plane_lenx=10  plane_leny=10  plane_depth=0.0001  force_law=Linear  k_contact=6e4  b_contact=2e2  pen_full_damp_F=1e-4  pen_exponent=1  custom_param_1=1  custom_param_2=1  friction_law=Stick-Slip Continuous  mu_kinetic=0.5  mu_static=0.7  v_thr=0.1  vis_on=on  vis_opc_en=0  vis_len_plaBz=0.0001  vis_clr=[0.9 0.2 0.2]  vis_opc=0.7
  Midfoot to Heel : sm_lib/Frames and Transforms/Rigid Transform  TranslationMethod=Cartesian  TranslationStandardOffset=0  TranslationLengthUnit=m  TranslationStandardAxis=+Z  TranslationCartesianOffset=[-0.08; 0; 0]  TranslationROffset=0  TranslationROffsetUnits=m  TranslationZOffset=0  TranslationZOffsetUnits=m  TranslationThetaOffset=0  TranslationThetaOffsetUnits=deg  RotationMethod=None  RotationAngleUnits=deg  RotationStandardAxis=+Z  RotationAngle=0.0  RotationArbitraryAxis=[0 0 1]  FollAlignAxisA=+X  BaseAlignAxisA=+Y  FollAlignAxisB=+Y  BaseAlignAxisB=+Z  RotationSequenceAxes=FollowerAxes  RotationSequence=XYZ  RotationSequenceAngles=[-90 0 0]  RotationSequenceAnglesUnits=deg  RotationMatrix=[1 0 0; 0 1 0; 0 0 1]
  Midfoot to Toe : sm_lib/Frames and Transforms/Rigid Transform  TranslationMethod=Cartesian  TranslationStandardOffset=0  TranslationLengthUnit=m  TranslationStandardAxis=+Z  TranslationCartesianOffset=[0.08; 0; 0]  TranslationROffset=0  TranslationROffsetUnits=m  TranslationZOffset=0  TranslationZOffsetUnits=m  TranslationThetaOffset=0  TranslationThetaOffsetUnits=deg  RotationMethod=None  RotationAngleUnits=deg  RotationStandardAxis=+Z  RotationAngle=0.0  RotationArbitraryAxis=[0 0 1]  FollAlignAxisA=+X  BaseAlignAxisA=+Y  FollAlignAxisB=+Y  BaseAlignAxisB=+Z  RotationSequenceAxes=FollowerAxes  RotationSequence=XYZ  RotationSequenceAngles=[0 0 0]  RotationSequenceAnglesUnits=deg  RotationMatrix=[1 0 0; 0 1 0; 0 0 1]
  Revolute Joint : sm_lib/Joints/Revolute Joint  SenseConstraintForce=off  SenseConstraintForceX=off  SenseConstraintForceY=off  SenseConstraintForceZ=off  SenseConstraintTorque=off  SenseConstraintTorqueX=off  SenseConstraintTorqueY=off  SenseConstraintTorqueZ=off  SenseTotalForce=off  SenseTotalForceX=off  SenseTotalForceY=off  SenseTotalForceZ=off  SenseTotalTorque=off  SenseTotalTorqueX=off  SenseTotalTorqueY=off  SenseTotalTorqueZ=off  CompositeWrenchDir=FollowerOnBase  CompositeWrenchFrame=BaseFrame  EquilibriumPosition=0  EquilibriumPositionUnits=deg  SpringStiffness=0  SpringStiffnessUnits=N*m/deg  DampingCoefficient=0  DampingCoefficientUnits=N*m/(deg/s)  TorqueActuationMode=NoTorque  MotionActuationMode=ComputedMotion  SensePosition=off  SenseVelocity=off  SenseAcceleration=off  SenseTorqueForce=off  PositionTargetSpecify=on  PositionTargetPriority=Low  PositionTargetValue=cassieEtherCatData.leftFootDrive.inputs.position  PositionTargetValueUnits=rad  VelocityTargetSpecify=on  VelocityTargetPriority=High  VelocityTargetValue=0  VelocityTargetValueUnits=rad/s
  Toe Ground Contact : Contact_Forces_Lib/3D/Sphere to Plane Force  sphere_rad=0.01  plane_lenx=10  plane_leny=10  plane_depth=0.0001  force_law=Linear  k_contact=6e4  b_contact=2e2  pen_full_damp_F=1e-4  pen_exponent=1  custom_param_1=1  custom_param_2=1  friction_law=Stick-Slip Continuous  mu_kinetic=0.5  mu_static=0.7  v_thr=0.1  vis_on=on  vis_opc_en=0  vis_len_plaBz=0.0001  vis_clr=[0.9 0.2 0.2]  vis_opc=0.7
  World Frame : sm_lib/Frames and Transforms/World Frame
  Tarsus : PMIOPort  Port=1  Side=Left
  Plantar Rod : PMIOPort  Port=2  Side=Left
  connections:
  Revolute Joint/LConn1 -- Tarsus/RConn1
  Foot to Plantar Rod/LConn1 -- Foot/RConn1 -- Revolute Joint/RConn1 -- Foot to Midfoot/LConn1
  Plantar Rod/RConn1 -- Foot to Plantar Rod/RConn1
  Toe Ground Contact/LConn1 -- Midfoot to Toe/RConn1
  Heel Ground Contact/LConn1 -- Midfoot to Heel/RConn1
  Foot to Midfoot/RConn1 -- Midfoot to Heel/LConn1 -- Midfoot to Toe/LConn1
  Heel Ground Contact/RConn1 -- Toe Ground Contact/RConn1 -- World Frame/RConn1

== system SimulationLibrary/Heel Spring ==
  End Center to Pivot : sm_lib/Frames and Transforms/Rigid Transform  TranslationMethod=Cartesian  TranslationStandardOffset=0  TranslationLengthUnit=m  TranslationStandardAxis=+Z  TranslationCartesianOffset=[0.11877, -0.01, 0]  TranslationROffset=0  TranslationROffsetUnits=m  TranslationZOffset=0  TranslationZOffsetUnits=m  TranslationThetaOffset=0  TranslationThetaOffsetUnits=deg  RotationMethod=None  RotationAngleUnits=deg  RotationStandardAxis=+Z  RotationAngle=0.0  RotationArbitraryAxis=[0 0 1]  FollAlignAxisA=+X  BaseAlignAxisA=+Y  FollAlignAxisB=+Y  BaseAlignAxisB=+Z  RotationSequenceAxes=FollowerAxes  RotationSequence=XYZ  RotationSequenceAngles=[-90 0 0]  RotationSequenceAnglesUnits=deg  RotationMatrix=[1 0 0; 0 1 0; 0 0 1]
  Heel Spring Solid : sm_lib/Body Elements/Solid  InertiaType=Custom  Mass=0.1259  MassUnits=kg  CenterOfMass=[80.97; 2.23; -0.0385]/1000  CenterOfMassUnits=m  MomentsOfInertia=[30.16; 1049; 1028]/1000000  MomentsOfInertiaUnits=kg*m^2  ProductsOfInertia=[-0.0557; 0.575; 15.28]/1000000  ProductsOfInertiaUnits=kg*m^2  DensityBased=on  Density=1000  DensityUnits=kg/m^3  DoExposeReferenceFrame=on  SerializedFrames=<Frames/>  GraphicType=None  MarkerShape=Sphere  MarkerSize=10  GraphicVisPropType=SimpleVisualProperties  GraphicDiffuseColor=[0.5 0.5 0.5]  GraphicSpecularColor=[0.5 0.5 0.5 1.0]  GraphicAmbientColor=[0.15 0.15 0.15 1.0]  GraphicEmissiveColor=[0.0 0.0 0.0 1.0]  GraphicShininess=75  GraphicOpacity=1.0  GeometryShape=Brick  RectangleSize=[1 1]  RectangleSizeUnits=m  BrickDimensions=[1 1 1]  BrickDimensionUnits=m  CylinderRadius=1  CylinderRadiusUnits=m  CylinderLength=1  CylinderLengthUnits=m  SphereRadius=1  SphereRadiusUnits=m  EllipsoidRadii=[1 1 1]  EllipsoidRadiiUnits=m  ExtrusionCrossSection=[1 1; -1 1; -1 -1; 1 -1]  ExtrusionCrossSectionUnits=m  ExtrusionLength=1  ExtrusionLengthUnits=m  PolygonNumSides=3  PolygonOuterRadius=1  PolygonOuterRadiusUnits=m  ExtGeomFileType=STEP  ExtGeomFileUnits=m  RevolutionCrossSection=[1 1; 1 -1; 2 -1; 2 1]  RevolutionCrossSectionUnits=m  RevolutionExtent=Full  RevolutionAngle=180  RevolutionAngleUnits=deg
  Revolute Joint : sm_lib/Joints/Revolute Joint  SenseConstraintForce=off  SenseConstraintForceX=off  SenseConstraintForceY=off  SenseConstraintForceZ=off  SenseConstraintTorque=off  SenseConstraintTorqueX=off  SenseConstraintTorqueY=off  SenseConstraintTorqueZ=off  SenseTotalForce=off  SenseTotalForceX=off  SenseTotalForceY=off  SenseTotalForceZ=off  SenseTotalTorque=off  SenseTotalTorqueX=off  SenseTotalTorqueY=off  SenseTotalTorqueZ=off  CompositeWrenchDir=FollowerOnBase  CompositeWrenchFrame=BaseFrame  EquilibriumPosition=0  EquilibriumPositionUnits=rad  SpringStiffness=CassieParameters.springStiffness(2)  SpringStiffnessUnits=N*m/rad  DampingCoefficient=0  DampingCoefficientUnits=N*m/(rad/s)  TorqueActuationMode=NoTorque  MotionActuationMode=ComputedMotion  SensePosition=off  SenseVelocity=off  SenseAcceleration=off  SenseTorqueForce=off  PositionTargetSpecify=on  PositionTargetPriority=High  PositionTargetValue=0  PositionTargetValueUnits=rad  VelocityTargetSpecify=on  VelocityTargetPriority=High  VelocityTargetValue=0  VelocityTargetValueUnits=rad/s
  Tarsus : PMIOPort  Port=1  Side=Left
  Achilles : PMIOPort  Port=2  Side=Right
  connections:
  End Center to Pivot/RConn1 -- Achilles/RConn1
  Revolute Joint/LConn1 -- Tarsus/RConn1
  End Center to Pivot/LConn1 -- Revolute Joint/RConn1 -- Heel Spring Solid/RConn1

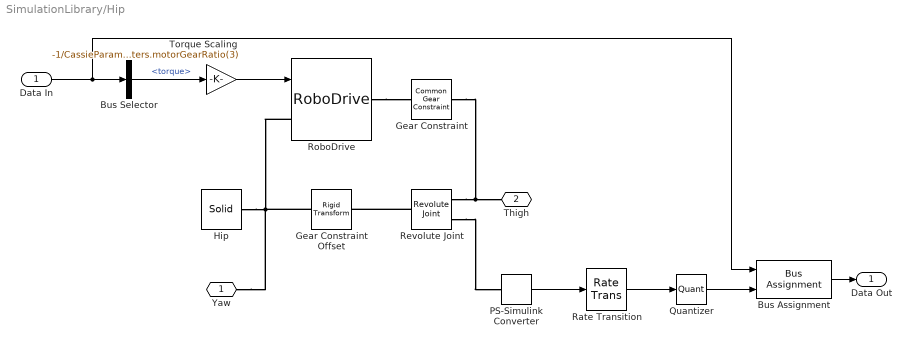
== system SimulationLibrary/Hip ==
  Data In : Inport  OutDataTypeStr=Bus: cassieEtherCatBus
  Bus Assignment : BusAssignment  AssignedSignals=leftHipDrive.inputs.position
  Bus Selector : BusSelector  OutputSignals=leftHipDrive.outputs.torque
  Gear Constraint : sm_lib/Gears and Couplings/Gears/Common Gear Constraint  GearType=External  SpecificationType=CenterDistanceRatio  CenterDistance=1e-6  CenterDistanceUnits=m  GearRatio=CassieParameters.motorGearRatio(3)  BaseGearRadius=10.0  BaseGearRadiusUnits=cm  FollGearRadius=10.0  FollGearRadiusUnits=cm  AssemblyGearRotation=Free
  Gear Constraint Offset : sm_lib/Frames and Transforms/Rigid Transform  TranslationMethod=StandardAxis  TranslationStandardOffset=1e-6  TranslationLengthUnit=m  TranslationStandardAxis=+Y  TranslationCartesianOffset=[0 0 0]  TranslationROffset=0  TranslationROffsetUnits=m  TranslationZOffset=0  TranslationZOffsetUnits=m  TranslationThetaOffset=0  TranslationThetaOffsetUnits=deg  RotationMethod=None  RotationAngleUnits=deg  RotationStandardAxis=+Z  RotationAngle=0.0  RotationArbitraryAxis=[0 0 1]  FollAlignAxisA=+X  BaseAlignAxisA=+Y  FollAlignAxisB=+Y  BaseAlignAxisB=+Z  RotationSequenceAxes=FollowerAxes  RotationSequence=XYX  RotationSequenceAngles=[0 0 0]  RotationSequenceAnglesUnits=deg  RotationMatrix=[1 0 0; 0 1 0; 0 0 1]
  Hip : sm_lib/Body Elements/Solid  InertiaType=Custom  Mass=1.171  MassUnits=kg  CenterOfMass=[-55.72; 0; 0.01]/1000  CenterOfMassUnits=m  MomentsOfInertia=[842; 6076; 6436]/1000000  MomentsOfInertiaUnits=kg*m^2  ProductsOfInertia=[-0.04; -0.6251; 0.2462]/1000000  ProductsOfInertiaUnits=kg*m^2  DensityBased=on  Density=1000  DensityUnits=kg/(m^3)  DoExposeReferenceFrame=on  SerializedFrames=<Frames/>  GraphicType=FromGeometry  MarkerShape=Sphere  MarkerSize=10  MarkerSizeUnits=m  GraphicVisPropType=AdvancedVisualProperties  GraphicDiffuseColor=simulationParameters.diffuseColor  GraphicSpecularColor=simulationParameters.specularColor  GraphicAmbientColor=simulationParameters.ambientColor  GraphicEmissiveColor=simulationParameters.emissiveColor  GraphicShininess=simulationParameters.shininess  GraphicOpacity=1  GeometryShape=FromFile  RectangleSize=[1 1]  RectangleSizeUnits=m  BrickDimensions=[0.15 0.15 0.2]  BrickDimensionUnits=m  CylinderRadius=0.05  CylinderRadiusUnits=m  CylinderLength=0.1  CylinderLengthUnits=m  SphereRadius=1  SphereRadiusUnits=m  EllipsoidRadii=[1 1 1]  EllipsoidRadiiUnits=m  ExtrusionCrossSection=[1 1; -1 1; -1 -1; 1 -1]  ExtrusionCrossSectionUnits=m  ExtrusionLength=1  ExtrusionLengthUnits=m  PolygonNumSides=3  PolygonOuterRadius=1  PolygonOuterRadiusUnits=m  ExtGeomFileType=STL  ExtGeomFileName=left_hip.stl  ExtGeomFileUnits=m  RevolutionCrossSection=[1 1; 1 -1; 2 -1; 2 1]  RevolutionCrossSectionUnits=m  RevolutionExtent=Full  RevolutionAngle=180  RevolutionAngleUnits=deg
  PS-Simulink Converter : nesl_utility/PS-Simulink Converter  PhysicalDomain=network_engine_domain  SubClassName=ps_output  LeftPortType=input  RightPortType=output  PseudoPeriodic=off  Frequencies=[]  Unit=rad  AffineConversion=off
  Quantizer : Quantizer  QuantizationInterval=(2*pi)/(CassieParameters.motorEncoderTicks(3)*CassieParameters.motorGearRatio(3))
  Rate Transition : RateTransition  Deterministic=off  OutPortSampleTime=CassieParameters.etherCatSampleTime
  Revolute Joint : sm_lib/Joints/Revolute Joint  SenseConstraintForce=off  SenseConstraintForceX=off  SenseConstraintForceY=off  SenseConstraintForceZ=off  SenseConstraintTorque=off  SenseConstraintTorqueX=off  SenseConstraintTorqueY=off  SenseConstraintTorqueZ=off  SenseTotalForce=off  SenseTotalForceX=off  SenseTotalForceY=off  SenseTotalForceZ=off  SenseTotalTorque=off  SenseTotalTorqueX=off  SenseTotalTorqueY=off  SenseTotalTorqueZ=off  CompositeWrenchDir=FollowerOnBase  CompositeWrenchFrame=BaseFrame  EquilibriumPosition=0  EquilibriumPositionUnits=rad  SpringStiffness=0  SpringStiffnessUnits=N*m/rad  DampingCoefficient=CassieParameters.motorViscousFrictionCoefficient(3)  DampingCoefficientUnits=N*m/(rad/s)  TorqueActuationMode=NoTorque  MotionActuationMode=ComputedMotion  SensePosition=on  SenseVelocity=off  SenseAcceleration=off  SenseTorqueForce=off  PositionTargetSpecify=on  PositionTargetPriority=High  PositionTargetValue=cassieEtherCatData.leftHipDrive.inputs.position  PositionTargetValueUnits=rad  VelocityTargetSpecify=on  VelocityTargetPriority=High  VelocityTargetValue=0  VelocityTargetValueUnits=rad/s
  RoboDrive : SimulationLibrary/RoboDrive  model=115x25
  Torque Scaling : Gain  Gain=-1/CassieParameters.motorGearRatio(3)
  Yaw : PMIOPort  Port=1  Side=Left
  Thigh : PMIOPort  Port=2  Side=Right
  Data Out : Outport
  wires:
  Torque Scaling/1 -> RoboDrive/1
  Data In/1 -> Bus Selector/1, Bus Assignment/1
  Bus Assignment/1 -> Data Out/1
  Rate Transition/1 -> Quantizer/1
  Bus Selector/1 -> Torque Scaling/1  "<torque>"
  PS-Simulink Converter/1 -> Rate Transition/1
  Quantizer/1 -> Bus Assignment/2
  connections:
  Hip/RConn1 -- RoboDrive/LConn1 -- Yaw/RConn1 -- Gear Constraint Offset/LConn1
  Revolute Joint/LConn1 -- Gear Constraint Offset/RConn1
  RoboDrive/RConn1 -- Gear Constraint/LConn1
  Revolute Joint/RConn2 -- PS-Simulink Converter/LConn1
  Gear Constraint/RConn1 -- Revolute Joint/RConn1 -- Thigh/RConn1
